simulink model "mathtest"  (R2018a)
settings: Solver=FixedStepAuto  StartTime=0.0  StopTime=10.0  FixedStep=0.1  RelTol=1e-3
settings Model: Creator=paul  LastModifiedBy=paul

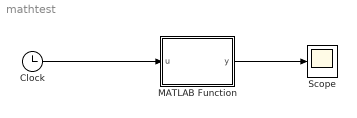
== system mathtest ==
  Clock : Clock
  MATLAB Function : MATLAB Function  TreatAsAtomicUnit=on
  Scope : Scope
  wires:
  Clock/1 -> MATLAB Function/1(u)
  MATLAB Function/1(y) -> Scope/1

== matlab function mathtest/MATLAB Function ==
  data: u input; y output
function y = fcn(u)
coder.extrinsic('py.mathtest.sinu')

a = 0;
a = py.mathtest.sinu(u);

y = a;
